simulink model "SimulationOpenLoopModel"  (R2024a)
settings: Solver=FixedStepAuto  StartTime=0.0  StopTime=tFinal_s  FixedStep=deltaT_s  RelTol=1e-3
values from neighbouring files (symbols this model uses):
  K = 49    [Step01a_AnalyzeStepResponse.m]
  stepMagnitude = 1    [Step01a_AnalyzeStepResponse.m]
  stepTime_s = 5    [Step01a_AnalyzeStepResponse.m]
  Tambient_C = tempTC(10)    [Step01a_AnalyzeStepResponse.m]
undefined symbols (not defined in the file or in its folder): b
libraries: TemperatureControlLibrary x2
settings Model: Creator=chris  LastModifiedBy=chris

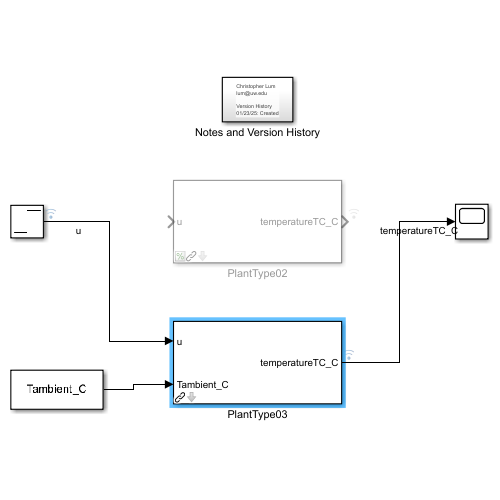
[thumbnail: Simulink's stored preview of the top-level diagram]
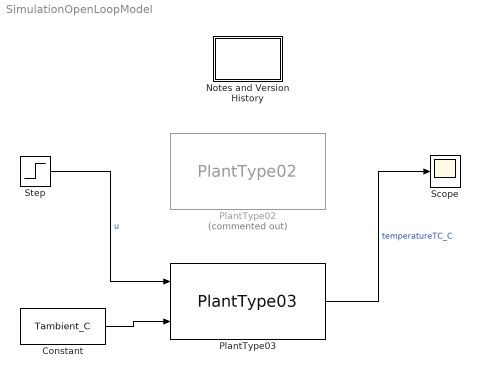
== system SimulationOpenLoopModel ==
  Constant : Constant  Value=Tambient_C
  Notes and Version History : Subsystem
  PlantType02 : TemperatureControlLibrary/PlantType02  Commented=on  a=a  b=b  T0=25
  PlantType03 : TemperatureControlLibrary/PlantType03  wn=wn  zeta=zeta  K=K  Tdelay_s=Tdelay_s
  Scope : Scope
  Step : Step  Time=stepTime_s  After=stepMagnitude  SampleTime=0
  wires:
  Step/1 -> PlantType03/1  "u"
  PlantType03/1 -> Scope/1  "temperatureTC_C"
  Constant/1 -> PlantType03/2

== system SimulationOpenLoopModel/Notes and Version History ==
  note: Christopher Lum
      | lum@uw.edu
      |
      | Version History
      | 01/23/25: Created
